simulink model "c_ep_approx"  (R2024b)
settings: Solver=VariableStepAuto  StartTime=0.0  StopTime=1000  RelTol=1e-3
settings Model: Creator=merlin  LastModifiedBy=merlin

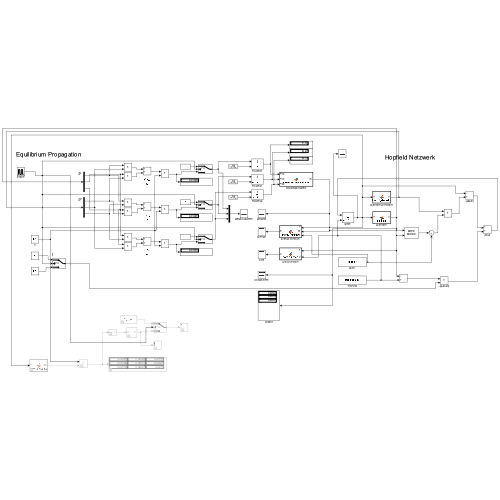
[thumbnail: Simulink's stored preview of the top-level diagram]
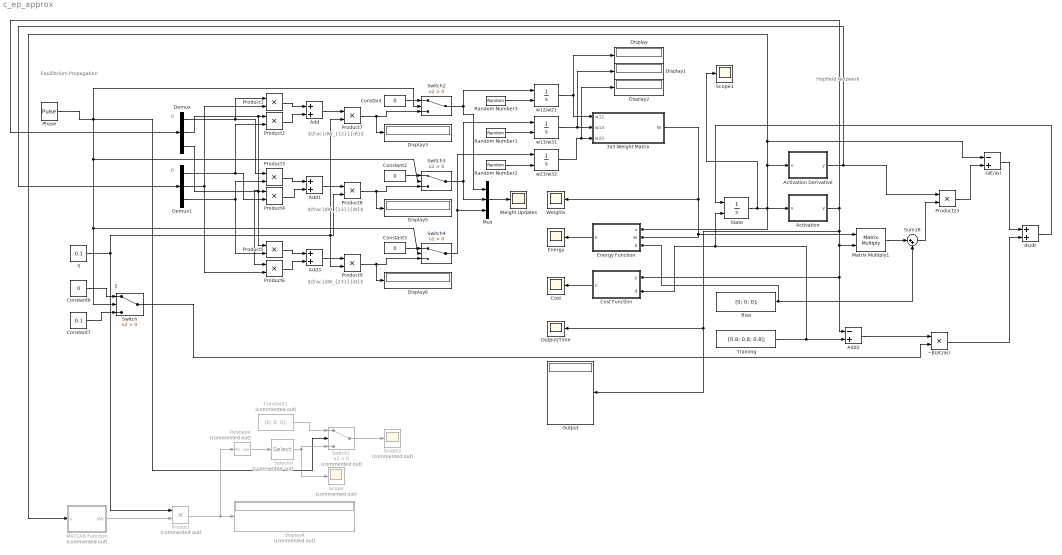
== system c_ep_approx ==
  note: ρ
  note: β
  note: Equilibrium Propagation
  note: Hopfield Netzwerk
  note: ρ′
  note: $\frac{dW_{12}}{dt}$
  note: $\frac{dW_{13}}{dt}$
  note: $\frac{dW_{23}}{dt}$
  -(∂E/∂s) : Sum  Inputs=-+
  3x3 Weight Matrix : MATLAB Function  TreatAsAtomicUnit=on
  Activation : MATLAB Function  TreatAsAtomicUnit=on
  Activation Derivative : MATLAB Function  TreatAsAtomicUnit=on
  Add : Sum
  Add1 : Sum
  Add2 : Sum  Inputs=-+
  Add3 : Sum
  Bias : Constant  Value=[0; 0; 0];  VectorParams1D=off
  Constant{,2..3,6} (4 alike) : Constant  Value=0
  Constant1 : Constant  Commented=on  Value=[0; 0; 0];
  Constant7 : Constant  Value=0.1
  Cost : Scope
  Cost Function : MATLAB Function  TreatAsAtomicUnit=on
  Demux : Demux  Outputs=3
  Demux1 : Demux  Outputs=3
  Display{,1..3,5..6} (6 alike) : Display
  Display4 : Display  Commented=on
  Energy : Scope
  Energy Function : MATLAB Function  TreatAsAtomicUnit=on
  MATLAB Function : MATLAB Function  Commented=on  TreatAsAtomicUnit=on
  Matrix Multiply1 : Product  Multiplication=Matrix(*)
  Mux : Mux  Inputs=3
  Output : Display
  Output/Time : Scope
  Phase : DiscretePulseGenerator  PulseType=Time based  Period=1000  PulseWidth=5
  Product : Product  Commented=on
  Product{1..9,23} (10 alike) : Product
  Random Number1 : RandomNumber  Seed=13  SampleTime=0.1
  Random Number2 : RandomNumber  Seed=23  SampleTime=0.1
  Random Number3 : RandomNumber  Seed=12  SampleTime=0.1
  Reshape : Reshape  Commented=on
  Scope : Scope  Commented=on
  Scope1 : Scope
  Scope2 : Scope  Commented=on
  Selector : Selector  Commented=on  IndexMode=Zero-based  InputPortWidth=9  IndexOptions=Index vector (dialog)  Indices=[1 2 5]  OutputSizes=1
  State : Integrator  InitialConditionSource=external
  Sum18 : Sum  Inputs=|++
  Switch{,2..4} (4 alike) : Switch  Criteria=u2 > Threshold  SaturateOnIntegerOverflow=off  InputSameDT=off
  Switch1 : Switch  Commented=on  Criteria=u2 > Threshold  SaturateOnIntegerOverflow=off  InputSameDT=off
  Training : Constant  Value=[0.8; 0.8; 0.8];  VectorParams1D=off
  Weight Updates : Scope
  Weights : Scope
  ds/dt : Sum
  w12/w21 : Integrator  InitialConditionSource=external
  w13/w31 : Integrator  InitialConditionSource=external
  w23/w32 : Integrator  InitialConditionSource=external
  η : Constant  Value=0.1
  −β(∂C/∂s) : Product
  wires:
  Constant6/1 -> Switch/1
  Constant7/1 -> Switch/3
  Phase/1 -> Switch4/2, Switch/2, Switch3/2, Switch2/2, Switch1/2
  Product23/1 -> -(∂E/∂s)/2
  Energy Function/1(E) -> Energy/1
  −β(∂C/∂s)/1 -> ds/dt/2
  Cost Function/1(C) -> Cost/1
  3x3 Weight Matrix/1(W) -> Weights/1, Energy Function/2(W), Matrix Multiply1/1
  Bias/1 -> Sum18/2, Energy Function/3(b)
  w12/w21/1 -> 3x3 Weight Matrix/1(w12), Display/1
  ds/dt/1 -> State/1
  Training/1 -> Cost Function/2(d), State/2, Add2/2
  -(∂E/∂s)/1 -> ds/dt/1
  Add2/1 -> −β(∂C/∂s)/1
  Sum18/1 -> Product23/2
  Matrix Multiply1/1 -> Sum18/1
  Activation Derivative/1(y) -> Demux1/1, Product23/1
  Constant1/1 -> Switch1/1
  Reshape/1 -> Selector/1
  State/1 -> Scope1/1, Activation/1(u), Energy Function/1(u), MATLAB Function/1(u), -(∂E/∂s)/1, Activation Derivative/1(u)
  Selector/1 -> Switch1/3, Scope/1
  MATLAB Function/1(dW) -> Product/2
  Product/1 -> Reshape/1, Display4/1
  Activation/1(y) -> Add2/1, Cost Function/1(y), Matrix Multiply1/2, Output/1, Output/Time/1, Demux/1
  Switch/1 -> −β(∂C/∂s)/2
  Random Number3/1 -> w12/w21/2
  Random Number1/1 -> w13/w31/2
  Random Number2/1 -> w23/w32/2
  w13/w31/1 -> Display1/1, 3x3 Weight Matrix/2(w13)
  w23/w32/1 -> Display2/1, 3x3 Weight Matrix/3(w23)
  η/1 -> Product7/2, Product8/2, Product9/2, Product/1
  Switch1/1 -> Scope2/1
  Product1/1 -> Add/1
  Product2/1 -> Add/2
  Product3/1 -> Add1/1
  Product6/1 -> Add3/2
  Product5/1 -> Add3/1
  Constant/1 -> Switch2/1
  Constant2/1 -> Switch3/1
  Constant3/1 -> Switch4/1
  Product4/1 -> Add1/2
  Demux1/2 -> Product6/2, Product1/2
  Demux1/1 -> Product4/2, Product2/2
  Demux1/3 -> Product5/2, Product3/2
  Switch2/1 -> Mux/1, w12/w21/1
  Switch3/1 -> Mux/2, w13/w31/1
  Switch4/1 -> w23/w32/1, Mux/3
  Add/1 -> Product7/1
  Product7/1 -> Display3/1, Switch2/3
  Add1/1 -> Product8/1
  Add3/1 -> Product9/1
  Product8/1 -> Display5/1, Switch3/3
  Product9/1 -> Display6/1, Switch4/3
  Mux/1 -> Weight Updates/1
  Demux/1 -> Product3/1, Product1/1
  Demux/2 -> Product5/1, Product2/1
  Demux/3 -> Product6/1, Product4/1

== matlab function c_ep_approx/3x3 Weight Matrix ==
  data: w12 input; W output; w13 input; w23 input
function W = create3x3WeightMatrix(w12, w13, w23)
    W = [0,    w12,  w13;
         w12,  0,    w23;
         w13,  w23,  0];
end

== matlab function c_ep_approx/Energy Function ==
  data: u input; E output; W input; b input
function E = energy_function(u, W, b)
    rho = @(x) 1 ./ (1 + exp(-x));

    E = (1/2) * sum(u.^2) ...
        - (1/2) * sum(sum(W .* (rho(u) * rho(u)')))
        - sum(b .* rho(u));
end

== matlab function c_ep_approx/MATLAB Function ==
  data: u input; dW output
function dW = weight_update(u)
% u: Vector of neuron states
% W: Current weight matrix
% dW: Rate of change of weights

% Define sigmoid function
rho = @(x) 1 ./ (1 + exp(-x));
% rho = @(x) 2 ./ (1 + exp(-x)) - 1;

% Compute sigmoid values for each neuron
rho_u = rho(u);

% Compute the derivative of the sigmoid (rho_dot)
rho_dot = rho_u .* (1 - rho_u);
% rho_dot = 2 .* rho_u .* (1 - rho_u);


% Compute weight update (Hebbian-like rule)
dW = rho_dot * rho_u' + rho_u * rho_dot';

end

== matlab function c_ep_approx/Activation Derivative ==
  data: u input; y output
function y = sigmoid_derivative(u)
% Activation Function: Logistic Function
sigmoid = 1 ./ (1 + exp(-u));
y = sigmoid .* (1 - sigmoid);

% Activation Function: Scaled Logistic Function
% sigmoid = 1 ./ (1 + exp(-u));
% y = 2 .* sigmoid .* (1 - sigmoid);

% Activation Function: tanh
% y = 1 - tanh(u).^2;

% Activation Function: ReLU
% y = double(u > 0);
end

== matlab function c_ep_approx/Activation ==
  data: u input; y output
function y = sigmoid(u)
% Activation Function: Logistic Function
y = 1 ./ (1 + exp(-u));

% Activation Function: Scaled Logistic Function
% y = 2 .* 1 ./ (1 + exp(-u)) - 1;

% Activation Function: tanh
% y = tanh(u);

% Activation Function: ReLU
% y = max(u, 0);
end

== matlab function c_ep_approx/Cost Function ==
  data: y input; C output; d input
function C = cost_function(y, d)
    C = 0.5 * sum((y - d).^2);
end
